simulink model "superProgram"  (R2014b)
settings: Solver=FixedStepDiscrete  StartTime=0.0  StopTime=10.0  RelTol=1e-3
libraries: c2833xlib x18, c280xlib x6, simulink x1
(part 2 of 2)

== stateflow chart superProgram/stackerController ==
  state startingSequence [parallel]
    settings: executionOrder=1
    state prepareStacker
      entry:
      stackerMode = int16(0);
      speedCenterPivotTable = uint16(0);
      directionCenterPivotTable = true;
      speedPaternoster = uint16(0);
      directionPaternoster = true;
      speedKicker = uint16(0);
      directionKicker = true;
      speedTipper = uint16(0);
      directionTipper = true;
    state operationMode
    state waitingForButtonRelaseToStartSuperProgram
    (default) -> prepareStacker
    prepareStacker -> waitingForButtonRelaseToStartSuperProgram : [powerButton == true]
    waitingForButtonRelaseToStartSuperProgram -> operationMode : [powerButton == false] {send(sorting.START); send(timer.START);}
  note: add all motors to prepareStacker
  state counterFromLightBarrierCrossed [parallel]
    settings: executionOrder=3
    state start
      entry: count = uint32(0);
    state highLevel
    state lowLevel
      entry: count = count + 1;
    counterFromLightBarrierCrossed.lowLevel -> counterFromLightBarrierCrossed.highLevel : [encoderPaternoster == true]
    (default) -> counterFromLightBarrierCrossed.start
    counterFromLightBarrierCrossed.start -> counterFromLightBarrierCrossed.lowLevel : [encoderPaternoster == true]
    counterFromLightBarrierCrossed.highLevel -> counterFromLightBarrierCrossed.lowLevel : [encoderPaternoster == false]
    counterFromLightBarrierCrossed -> counterFromLightBarrierCrossed.start : RESET
  state timer [parallel]
    settings: executionOrder=2
    state startReturningBlocksFromRecervoir
      entry: send(sorting.STARTRESORTING);
    state start
    state inactive
    inactive -> startReturningBlocksFromRecervoir : after(latestPointInTimeToAcceptBlockDelivery,sec)
    (default) -> timer.start
    timer.start -> inactive : START
  state statusLED [parallel]
    settings: executionOrder=7
    state LED_1 [parallel]
      settings: executionOrder=1
      state off
        entry: statusLED_1 = false;
      state flash
        entry: statusLED_1 = true;
      state on
        entry: statusLED_1 = true;
      (default) -> statusLED.LED_1.off
      statusLED.LED_1.off -> statusLED.LED_1.on [order 1] : ON
      statusLED.LED_1.on -> statusLED.LED_1.off : OFF
      statusLED.LED_1.flash -> statusLED.LED_1.off : after(300,msec)
      statusLED.LED_1.off -> statusLED.LED_1.flash [order 2] : FLASH
    state LED_2 [parallel]
      settings: executionOrder=2
      state off
        entry: statusLED_2 = false;
      state flash
        entry: statusLED_2 = true;
      state on
        entry: statusLED_2 = true;
      (default) -> statusLED.LED_2.off
      statusLED.LED_2.off -> statusLED.LED_2.on [order 1] : ON
      statusLED.LED_2.on -> statusLED.LED_2.off : OFF
      statusLED.LED_2.flash -> statusLED.LED_2.off : after(300,msec)
      statusLED.LED_2.off -> statusLED.LED_2.flash [order 2] : FLASH
    state LED_3 [parallel]
      settings: executionOrder=3
      state off
        entry: statusLED_3 = false;
      state flash
        entry: statusLED_3 = true;
      state on
        entry: statusLED_3 = true;
      (default) -> statusLED.LED_3.off
      statusLED.LED_3.off -> statusLED.LED_3.on [order 1] : ON
      statusLED.LED_3.on -> statusLED.LED_3.off : OFF
      statusLED.LED_3.flash -> statusLED.LED_3.off : after(300,msec)
      statusLED.LED_3.off -> statusLED.LED_3.flash [order 2] : FLASH
    state LED_4 [parallel]
      settings: executionOrder=4
      state off
        entry: statusLED_4 = false;
      state flash
        entry: statusLED_4 = true;
      state on
        entry: statusLED_4 = true;
      (default) -> statusLED.LED_4.off
      statusLED.LED_4.off -> statusLED.LED_4.on [order 1] : ON
      statusLED.LED_4.on -> statusLED.LED_4.off : OFF
      statusLED.LED_4.flash -> statusLED.LED_4.off : after(300,msec)
      statusLED.LED_4.off -> statusLED.LED_4.flash [order 2] : FLASH
    state LED_finish [parallel]
      settings: executionOrder=5
      state off
        entry: LED_finish = false;
      state flash
        entry: LED_finish = true;
      state on
        entry: LED_finish = true;
      (default) -> statusLED.LED_finish.off
      statusLED.LED_finish.off -> statusLED.LED_finish.on [order 1] : ON
      statusLED.LED_finish.on -> statusLED.LED_finish.off : OFF
      statusLED.LED_finish.flash -> statusLED.LED_finish.off : after(300,msec)
      statusLED.LED_finish.off -> statusLED.LED_finish.flash [order 2] : FLASH
  note: stackerModes:
      | 0: stackerPreparation
      | 1: stackerPositioning
      | 2: colorSorting firstDelivery
      | 3: waitingForSecondDelivery
      | 4: colorSorting secondDelivery
      | 5: resorting
      | 6: demolding
      | 7: finish
  state stackerModeStatusLED_controller [parallel]
    settings: executionOrder=8
    state stackerPreparation
      entry: statusLED.LED_1.FLASH;
      statusLED.LED_2.FLASH;
      statusLED.LED_3.FLASH;
      statusLED.LED_4.FLASH;
    state colorSortingFirstDelivery
      entry: statusLED.LED_1.ON;
    state waitingForSecondDelivery
      entry: statusLED.LED_2.ON;
    state changeMode
      entry: statusLED.LED_1.OFF;
      statusLED.LED_2.OFF;
      statusLED.LED_3.OFF;
      statusLED.LED_4.OFF;
    state colorSortingSecondDelivery
      entry: statusLED.LED_3.ON;
    state resorting
      entry: statusLED.LED_4.ON;
    state demolding
      entry: statusLED.LED_1.ON;
      statusLED.LED_2.ON;
      statusLED.LED_3.ON;
      statusLED.LED_4.ON;
    state finish
      entry: statusLED.LED_1.FLASH;
      statusLED.LED_2.FLASH;
      statusLED.LED_3.FLASH;
      statusLED.LED_4.FLASH;
    changeMode -> stackerPreparation [order 1] : [stackerMode == 0]
    stackerPreparation -> changeMode : after(1200,msec)
    changeMode -> colorSortingFirstDelivery [order 2] : [stackerMode == 2]
    colorSortingFirstDelivery -> changeMode : [stackerMode ~= 2]
    changeMode -> stackerModeStatusLED_controller.waitingForSecondDelivery [order 5] : [stackerMode ==3]
    stackerModeStatusLED_controller.waitingForSecondDelivery -> changeMode : [stackerMode ~= 3]
    changeMode -> colorSortingSecondDelivery [order 3] : [stackerMode == 4]
    colorSortingSecondDelivery -> changeMode : [stackerMode ~= 4]
    (default) -> changeMode
    stackerModeStatusLED_controller.finish -> changeMode : after(600,msec)
    changeMode -> stackerModeStatusLED_controller.finish [order 7] : [stackerMode == 7]
    stackerModeStatusLED_controller.demolding -> changeMode : [stackerMode ~= 6]
    changeMode -> stackerModeStatusLED_controller.demolding [order 6] : [stackerMode == 6]
    resorting -> changeMode : [stackerMode ~= 5]
    changeMode -> resorting [order 4] : [stackerMode == 5]
  state blockCounter [parallel]
    settings: executionOrder=4
    state start
      entry: blueBlocksPassed = uint16(0);
      redBlocksPassed = uint16(0);
    state idle
      entry: totalBlocksPassed = blueBlocksPassed + redBlocksPassed;
    blockCounter.idle -> blockCounter.idle [order 2] : ADDBLUEBLOCK
        | /{blueBlocksPassed = blueBlocksPassed + 1;
        | blueBlocksInRecervoir = blueBlocksInRecervoir + 1;}
    blockCounter.start -> blockCounter.idle
    (default) -> blockCounter.start : {blueBlocksInRecervoir = uint16(0);}
    blockCounter.idle -> blockCounter.idle [order 1] : ADDREDBLOCK
        | /{redBlocksPassed = redBlocksPassed + 1;}
    blockCounter -> blockCounter.start : RESET
  state sorting [parallel]
    settings: executionOrder=6
    state colorSorter
      entry: speedPaternoster = paternosterSpeed;
      state counterFromKick [parallel]
        settings: executionOrder=2
        state start
          entry: count = uint32(0);
        state highLevel
        state lowLevel
          entry: count = count + 1;
        sorting.colorSorter.counterFromKick.lowLevel -> sorting.colorSorter.counterFromKick.highLevel : [encoderPaternoster ==  true]
        (default) -> sorting.colorSorter.counterFromKick.start
        sorting.colorSorter.counterFromKick.start -> sorting.colorSorter.counterFromKick.lowLevel : [encoderPaternoster  == true]
        sorting.colorSorter.counterFromKick.highLevel -> sorting.colorSorter.counterFromKick.lowLevel : [encoderPaternoster == false]
        counterFromKick -> sorting.colorSorter.counterFromKick.start : RESET
      state kicker [parallel]
        settings: executionOrder=1
        state kicker_controller [parallel]
          settings: executionOrder=1
          state kick
            entry: send(colorSorter.counterFromKick.RESET);
            enqueuedBlocksToKick = enqueuedBlocksToKick -1;
            state startKickerMovement
              entry: directionKicker = false;
              speedKicker = uint16(100);
            state stopKickerMovement
              entry: speedKicker = uint16(0);
            (default) -> sorting.colorSorter.kicker.kicker_controller.kick.startKickerMovement
            sorting.colorSorter.kicker.kicker_controller.kick.startKickerMovement -> sorting.colorSorter.kicker.kicker_controller.kick.stopKickerMovement : [outerKickerButton == true]
          state idle
            entry: speedKicker = uint16(0);
          state reprepareKicker
            state startKickerMovement
              entry: speedKicker = uint16(100);
              directionKicker = true;
            state stopKickerMovement
              entry: speedKicker = uint16(0);
            (default) -> sorting.colorSorter.kicker.kicker_controller.reprepareKicker.startKickerMovement
            sorting.colorSorter.kicker.kicker_controller.reprepareKicker.startKickerMovement -> sorting.colorSorter.kicker.kicker_controller.reprepareKicker.stopKickerMovement : [innerKickerButton == true]
          (default) -> sorting.colorSorter.kicker.kicker_controller.idle
          sorting.colorSorter.kicker.kicker_controller.idle -> kick : [[counterFromLightBarrierCrossed.count >= positionOfStartingKickOut] && [enqueuedBlocksToKick > 0]]
          kick -> reprepareKicker : [colorSorter.counterFromKick.count >= freeSpaceTillReprepareKickerAfterKickOut]
          sorting.colorSorter.kicker.kicker_controller.reprepareKicker.stopKickerMovement -> sorting.colorSorter.kicker.kicker_controller.idle
      state lightBarrier_controller [parallel]
        settings: executionOrder=3
        state lightBarrierCrossed
          entry:
          send(colorSorter.color_controller.NEXTBLOCK);
        state idle
        state waitngForSecondMeasuring
          entry: send(counterFromLightBarrierCrossed.RESET);
        state secondMeasuring
        (default) -> sorting.colorSorter.lightBarrier_controller.idle : /{colorSorter.kicker.kicker_controller.enqueuedBlocksToKick =uint16( 0)}
        sorting.colorSorter.lightBarrier_controller.idle -> waitngForSecondMeasuring : [lightBarrierCrossed  == true]
        waitngForSecondMeasuring -> secondMeasuring : [counterFromLightBarrierCrossed.count >= 11]
        secondMeasuring -> lightBarrierCrossed [order 1] : [lightBarrierCrossed == true]
        secondMeasuring -> (junction 392) [order 2] : [lightBarrierCrossed == false]
        lightBarrierCrossed -> (junction 392) : [lightBarrierCrossed == false]
        (junction 392) -> sorting.colorSorter.lightBarrier_controller.idle
      state color_controller [parallel]
        settings: executionOrder=4
        note: blue block detected
        state blockToKick
          entry: colorSorter.kicker.kicker_controller.enqueuedBlocksToKick = colorSorter.kicker.kicker_controller.enqueuedBlocksToKick + 1;
        state blockNotToKick
        state waitingForBlockToPassColorSensor
        note: red block detected
        (default) -> blockNotToKick
        waitingForBlockToPassColorSensor -> (junction 198) [order 1] : [counterFromLightBarrierCrossed.count >= lastPositionToDetectBlockColor]
        (junction 198) -> blockToKick [order 1] : [shouldBeKicked == true]
            | /{send(blockCounter.ADDBLUEBLOCK);}
        blockNotToKick -> waitingForBlockToPassColorSensor : NEXTBLOCK /{shouldBeKicked = true;}
        (junction 198) -> (junction 199) [order 2] : [shouldBeKicked == false]
            | /{send(blockCounter.ADDREDBLOCK);}
        waitingForBlockToPassColorSensor -> waitingForBlockToPassColorSensor [order 2] : [colorSensor <= colorSorterBlockColorLimit] {shouldBeKicked = false;}
        (junction 199) -> blockNotToKick
        blockToKick -> (junction 199)
    state resorting_controller
      entry: stackerMode = int16(5);
      blocksInChute =  int16(6 + 1 - (blockCounter.totalBlocksPassed + hooksInPaternosterFromPaternosterIntakeToColorSensor));
      blocksInChute = blocksInChute + abs(blocksInChute) * int16([blocksInChute < 0]);
      blocksToTip = int16(blockCapacityFromTipperToPaternosterIntake) - blocksInChute;
      speedPaternoster = uint16(100);
      state chuteEnqueuing_controller [parallel]
        settings: executionOrder=1
        state idle
        state signalizeFreeSlotInChute
          exit: resorting_controller.blocksToTip = resorting_controller.blocksToTip + 1;
        sorting.resorting_controller.chuteEnqueuing_controller.idle -> signalizeFreeSlotInChute : [lightBarrierCrossed == true] {counterFromLightBarrierCrossed.RESET;}
        (default) -> sorting.resorting_controller.chuteEnqueuing_controller.idle
        signalizeFreeSlotInChute -> sorting.resorting_controller.chuteEnqueuing_controller.idle : [lightBarrierCrossed == false]
      state tipper_controller [parallel]
        settings: executionOrder=2
        state tip
          exit: resorting_controller.blocksToTip = resorting_controller. blocksToTip - 1;
          blockCounter.blueBlocksInRecervoir = blockCounter.blueBlocksInRecervoir - 1;
          state tipperMovement
            state tipperPreparation
              entry: directionTipper = false;
              speedTipper = tipperSpeed;
            state tipperPush
              entry: directionTipper = true;
              speedTipper = tipperSpeed;
            state tipperRemove
              entry: directionTipper = false;
            state tipperIdle
              entry: speedTipper = uint16(0);
            (default) -> tipperPreparation
            tipperPreparation -> tipperPush : [outerTipperButton == true]
            tipperPush -> tipperRemove : [innerTipperButton == true]
            tipperRemove -> sorting.resorting_controller.tipper_controller.tip.tipperMovement.tipperIdle : [outerTipperButton == true]
          (default) -> tipperMovement
        state tipperIdle
        sorting.resorting_controller.tipper_controller.tipperIdle -> tip : [resorting_controller.blocksToTip > 0]
        (default) -> sorting.resorting_controller.tipper_controller.tipperIdle
        sorting.resorting_controller.tipper_controller.tip.tipperMovement.tipperIdle -> sorting.resorting_controller.tipper_controller.tipperIdle
    state waitingForBlocksToReachTower
      state allBlocksFallenIntoTower
      state blockReachedTopOfPaternoster
        entry: speedPaternoster = uint16(0);
      state start
      (default) -> sorting.waitingForBlocksToReachTower.start
      blockReachedTopOfPaternoster -> allBlocksFallenIntoTower : after(timeBlockNeedsToFallIntoTowerFromTopOfPaternoster,msec)
      sorting.waitingForBlocksToReachTower.start -> blockReachedTopOfPaternoster : [counterFromLightBarrierCrossed.count >= distanceFromLightBarrierToTDCOfPaternoster]
    state stackerPositioning
      entry: stackerMode = int16(1);
      state stackerRotation
        state rotationMovement [parallel]
          settings: executionOrder=1
          state start
            entry: directionCenterPivotTable = [centerPivotTableRotationTargetAngle >= 0];
            targetTics = abs(centerPivotTableRotationTargetAngle/360*75*centerPivotTableTransitionRatio);
          state targetAngleReached
            entry: speedCenterPivotTable = uint16(0);
          state move
            entry: speedCenterPivotTable = centerPivotTableSpeed;
          (default) -> sorting.stackerPositioning.stackerRotation.rotationMovement.start
          move -> targetAngleReached : [rotationCounter.count >= targetTics]
          sorting.stackerPositioning.stackerRotation.rotationMovement.start -> move : {send(rotationCounter.RESET)}
        state rotationCounter [parallel]
          settings: executionOrder=2
          state start
            entry: count= uint32(0);
          state highLevel
          state lowLevel
            entry: count = count + 1;
          sorting.stackerPositioning.stackerRotation.rotationCounter.lowLevel -> sorting.stackerPositioning.stackerRotation.rotationCounter.highLevel : [encoderCenterPivotTable > 0]
          (default) -> sorting.stackerPositioning.stackerRotation.rotationCounter.start
          sorting.stackerPositioning.stackerRotation.rotationCounter.start -> sorting.stackerPositioning.stackerRotation.rotationCounter.lowLevel : [encoderCenterPivotTable > 0]
          sorting.stackerPositioning.stackerRotation.rotationCounter.highLevel -> sorting.stackerPositioning.stackerRotation.rotationCounter.lowLevel : [encoderCenterPivotTable == 0]
          rotationCounter -> sorting.stackerPositioning.stackerRotation.rotationCounter.start : RESET
      state towerPreparation
      note: to implement
      (default) -> stackerRotation
    state demolding
      entry: stackerMode = int16(6);
      state demoldingTower
      state removeStackerFromTargetArea
      (default) -> demoldingTower
      demoldingTower -> removeStackerFromTargetArea
    state finish
      entry: stackerMode = int16(7);
      statusLED.LED_finish.ON;
    state start
    note: to implement
    colorSorter -> resorting_controller [order 1] : [[stackerMode == 4] && [blockCounter.redBlocksPassed == 1]]
    resorting_controller -> waitingForBlocksToReachTower [order 1] : [blockCounter.totalBlocksPassed >= (6 + blockCounter.blueBlocksInRecervoir)]
    (default) -> sorting.start
    sorting.start -> stackerPositioning : START
    colorSorter -> resorting_controller [order 2] : [[stackerMode == 4] && [counterFromLightBarrierCrossed.count >= (toleratedBlocksForNotChangingStackerMode * distanceBetweenBlockHooks)]]
    resorting_controller -> waitingForBlocksToReachTower [order 2] : [counterFromLightBarrierCrossed.count >= (toleratedBlocksForNotChangingStackerMode * distanceBetweenBlockHooks)]
    colorSorter -> resorting_controller [order 3] : STARTRESORTING
    allBlocksFallenIntoTower -> sorting.demolding
    removeStackerFromTargetArea -> sorting.finish
    targetAngleReached -> colorSorter
  state mode_controller [parallel]
    settings: executionOrder=5
    state waitingForSecondDelivery
      entry: stackerMode = int16(3);
      send(blockCounter.RESET);
    state firstDelivery
      entry: stackerMode = int16(2);
    state start
    state secondDelivery
      entry: stackerMode = int16(4);
    firstDelivery -> mode_controller.waitingForSecondDelivery : [counterFromLightBarrierCrossed.count >= (minFreeHooksToChangeModeToWaitingForSecondDelivery * distanceBetweenBlockHooks)]
    mode_controller.waitingForSecondDelivery -> secondDelivery : [blockCounter.totalBlocksPassed >= 1]
    mode_controller.start -> firstDelivery : [blockCounter.totalBlocksPassed >= 1]
    (default) -> mode_controller.start
  data: count local uint32; blueBlocksPassed local uint16 [0..]; redBlocksPassed local uint16 [0..]; blueBlocksInRecervoir local uint16 [0..]; totalBlocksPassed local uint16 [0..]; count local uint32; enqueuedBlocksToKick local uint16 [0..2]; shouldBeKicked local boolean; blocksInChute local int16; blocksToTip local int16 [-6..15]; targetTics local single [0..]; count local uint32; powerButton input boolean; paternosterSpeed input uint16 [0..100]; centerPivotTableTransitionRatio input single [0..]; centerPivotTableSpeed input uint16 [0..100]; centerPivotTableRotationTargetAngle input single [-360..360]; encoderCenterPivotTable input boolean; latestPointInTimeToAcceptBlockDelivery input uint16 [0..]; speedCenterPivotTable output uint16 [0..100]; directionCenterPivotTable output boolean; speedPaternoster output uint16 [0..100]; directionPaternoster output boolean; speedKicker output uint16 [0..100]; directionKicker output boolean; speedTipper output uint16 [0..100]; directionTipper output boolean; encoderPaternoster input boolean; encoderKicker input boolean; lightBarrierCrossed input boolean; colorSensor input uint16 [0..4095]; colorSorterBlockColorLimit input uint16 [0..4095]; lastPositionToDetectBlockColor input uint32; positionOfStartingKickOut input uint32; distanceBetweenBlockHooks input uint16 [0..]; distanceFromPaternosterIntakeToLightBarrier input uint16 [0..]; distanceFromLightBarrierToTDCOfPaternoster input uint16 [0..]; freeSpaceTillReprepareKickerAfterKickOut input uint32; minFreeHooksToChangeModeToWaitingForSecondDelivery input uint16 [0..]; toleratedBlocksForNotChangingStackerMode input uint16 [0..]; kickerElongation input uint16 [0..]; hooksInPaternosterFromPaternosterIntakeToColorSensor input uint16 [0..]; statusLED_1 output boolean; statusLED_3 output boolean; blockCapacityFromTipperToPaternosterIntake input uint16 [0..]; timeBlockNeedsToFallIntoTowerFromTopOfPaternoster input uint16 [0..]; outerTipperButton input boolean; innerTipperButton input boolean; tipperSpeed input uint16 [0..100]; statusLED_2 output boolean; stackerMode local int16; statusLED_4 output boolean; outerKickerButton input boolean; innerKickerButton input boolean; LED_finish output boolean
  data centerPivotTableTransitionRatio settings: description=transition ration of the stacker center pivot plate
  data centerPivotTableRotationTargetAngle settings: description=rotation target angle for the center pivot table of the stacker
  data encoderCenterPivotTable settings: description=encoder signal of the center pivot table motor
  data speedCenterPivotTable settings: description=speedCenterPivotTable of the center pivot table motor
  data directionCenterPivotTable settings: description=direciton of the center pivot table motor
  data directionPaternoster settings: description=direciton of the center pivot table motor
  data directionKicker settings: description=direciton of the center pivot table motor
  data directionTipper settings: description=direciton of the center pivot table motor
  data encoderPaternoster settings: description=encoder signal from the paternoster
  data encoderKicker settings: description=encoder signal from the kicker
  data lightBarrierCrossed settings: description=bolean value if the light barrier is currently crossed
  data colorSensor settings: description=value from the ADC of the color sensor
  data colorSorterBlockColorLimit settings: description=color value limit between red and blue blocks which decides whether blocks should be kicked or not
  data lastPositionToDetectBlockColor settings: description=length from light barrier to last possible position for color detection of blocks in tics from encoder
  data positionOfStartingKickOut settings: description=length from light barrier to position where kicker starts off kicking out blocks in tics from encoder
  data freeSpaceTillReprepareKickerAfterKickOut settings: description=space to wait after the kick out of a block till kicker reprepares (crosses the drive lane again) in tics from encoder
  data kickerElongation settings: description=distance to move kicker in / out
  data statusLED_1 settings: description=status LED to signalize when the light barrier is currently crossed
  events: RESET local FUNCTION_CALL_EVENT; START local FUNCTION_CALL_EVENT; FLASH local FUNCTION_CALL_EVENT; ON local FUNCTION_CALL_EVENT; OFF local FUNCTION_CALL_EVENT; FLASH local FUNCTION_CALL_EVENT; ON local FUNCTION_CALL_EVENT; OFF local FUNCTION_CALL_EVENT; FLASH local FUNCTION_CALL_EVENT; ON local FUNCTION_CALL_EVENT; OFF local FUNCTION_CALL_EVENT; FLASH local FUNCTION_CALL_EVENT; ON local FUNCTION_CALL_EVENT; OFF local FUNCTION_CALL_EVENT; FLASH local FUNCTION_CALL_EVENT; ON local FUNCTION_CALL_EVENT; OFF local FUNCTION_CALL_EVENT; RESET local FUNCTION_CALL_EVENT; ADDBLUEBLOCK local FUNCTION_CALL_EVENT; ADDREDBLOCK local FUNCTION_CALL_EVENT; RESET local FUNCTION_CALL_EVENT; NEXTBLOCK local FUNCTION_CALL_EVENT; RESET local FUNCTION_CALL_EVENT; STARTRESORTING local FUNCTION_CALL_EVENT; START local FUNCTION_CALL_EVENT
